simulink model "Ej8"  (R2025a)
settings: Solver=VariableStepAuto  StartTime=0.0  StopTime=10  RelTol=1e-3
libraries: dspfdesign x2, commrandsrc3 x1
settings Model: Creator=Henry  LastModifiedBy=Henry

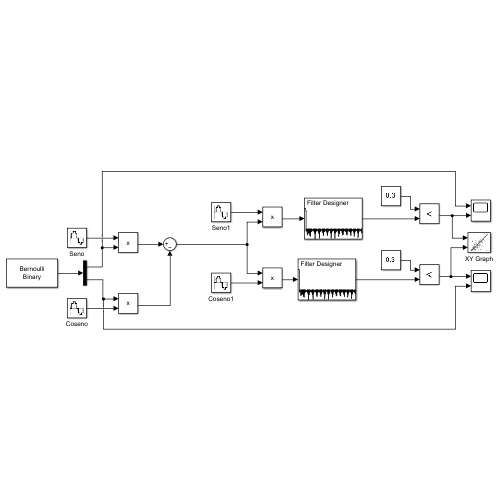
[thumbnail: Simulink's stored preview of the top-level diagram]
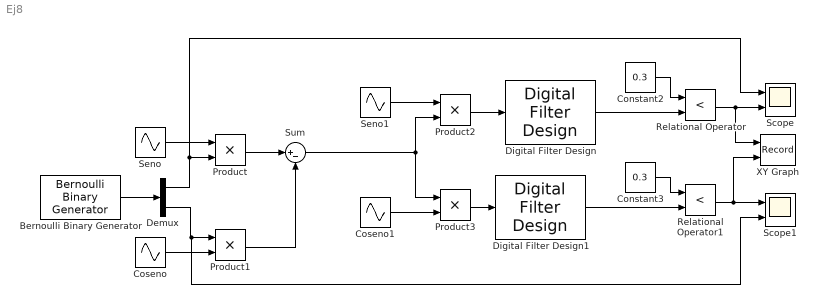
== system Ej8 ==
  Bernoulli Binary Generator : commrandsrc3/Bernoulli Binary Generator  ProbabilityOfZero=0.5  SeedSource=Auto  Seed=0  SampleTime=1  SamplesPerFrame=2  OutputDataType=double  SimulateUsing=Interpreted execution
  Constant2 : Constant  Value=0.3
  Constant3 : Constant  Value=0.3
  Coseno : Sin  Frequency=2*pi*100  Phase=pi/2  SampleTime=0.0001
  Coseno1 : Sin  Frequency=2*pi*100  Phase=-pi/2  SampleTime=0.0001
  Demux : Demux  Outputs=2
  Digital Filter Design : dspfdesign/Digital Filter Design  mwdsp_browser_bugfix_var=off
  Digital Filter Design1 : dspfdesign/Digital Filter Design  mwdsp_browser_bugfix_var=off
  Product{,1..3} (4 alike) : Product
  Relational Operator : RelationalOperator  Operator=<  OutDataTypeStr=boolean  RndMeth=Simplest  InputSameDT=off
  Relational Operator1 : RelationalOperator  Operator=<  OutDataTypeStr=boolean  RndMeth=Simplest  InputSameDT=off
  Scope : Scope  NumInputPorts=2
      settings: ActiveDisplayYMinimum=-1  ActiveDisplayYMaximum=1
  Scope1 : Scope  NumInputPorts=2
      settings: ActiveDisplayYMinimum=-1  ActiveDisplayYMaximum=1
  Seno : Sin  Frequency=2*pi*100  SampleTime=0.0001
  Seno1 : Sin  Frequency=2*pi*100  SampleTime=0.0001
  Sum : Sum  Inputs=|+-
  XY Graph : Record  NumPorts=2.0  FileSettingsInternal="{\"entries\":[{\"content\":{\"excelSettings\":{\"content\":{},\"type\":\"Streamout.ExcelSettings\"},\"parquetSettings\":{\"content\":{},\"type\":\"Streamout.ParquetSettings\"}},\"type\":\"Streamout.FileSettingStorage\",\"uuid\":\"\"}],\"packageUris\":[\"http:\\/\\/schema.mathworks.com\\/mf0\\/streamout_blocks\\/R2020a\"],\"version\":\"1.0\"}"  FrameSettings=[0, 0]  Layout=[1 1]  SignalsInternal="{\"entries\":[{\"content\":{\"signals\":[{\"content\":{\"blockPath\":[],\"dimensions\":[1],\"domain\":\"\",\"lineColor\":\"#a2142f\",\"plots\":[ 1 ],\"port\":1,\"sid\":[\"\"],\"signalID\":1,\"signalName\":\"Relational\\nOperator\"},\"type\":\"RecordBlkView.Signal\",\"uuid\":\"\"},{\"content\":{\"blockPath\":[],\"dimensions\":[1],\"domain\":\"\",\"lineColor\":\"#139fff\",\"plots\":[ 1 ],\"port\":2,\"sid\":[\"\"],\"signalID\":2,\"signalName\":\"Relational\\nOperator1\"},\"type\":\"RecordBlkView.Signal\",\"uuid\":\"\"}]},\"type\":\"RecordBlkView.InputSignals\",\"uuid\":\"\"}],\"packageUris\":[\"http:\\/\\/schema.mathworks.com\\/mf0\\/streamout_blocks\\/R2020a\"],\"version\":\"1.0\"}"  VisualizationBindings="{\"xyplotplugin\":{\"info\":[{\"series\":[{\"bindingParametersList\":[{\"parameter\":\"X-Axis\",\"signalID\":1,\"signalName\":\"Relational\\nOperator\"},{\"parameter\":\"Y-Axis\",\"signalID\":2,\"signalName\":\"Relational\\nOperator1\"}],\"seriesID\":0}],\"subplotID\":1}]}}"  CompatibilityTag=XY
  wires:
  Seno/1 -> Product/1
  Demux/1 -> Product/2, Scope/1
  Demux/2 -> Scope1/2, Product1/1
  Coseno/1 -> Product1/2
  Product/1 -> Sum/1
  Product1/1 -> Sum/2
  Coseno1/1 -> Product3/2
  Seno1/1 -> Product2/1
  Product2/1 -> Digital Filter Design/1
  Product3/1 -> Digital Filter Design1/1
  Digital Filter Design/1 -> Relational Operator/2
  Digital Filter Design1/1 -> Relational Operator1/2
  Constant2/1 -> Relational Operator/1
  Constant3/1 -> Relational Operator1/1
  Relational Operator/1 -> XY Graph/1, Scope/2
  Relational Operator1/1 -> XY Graph/2, Scope1/1
  Bernoulli Binary Generator/1 -> Demux/1
  Sum/1 -> Product3/1, Product2/2
